simulink model "lab2"  (R2022a)
settings: Solver=VariableStepAuto  StartTime=0.0  StopTime=10.0  RelTol=1e-3
settings Model: Creator=Комп  LastModifiedBy=Комп

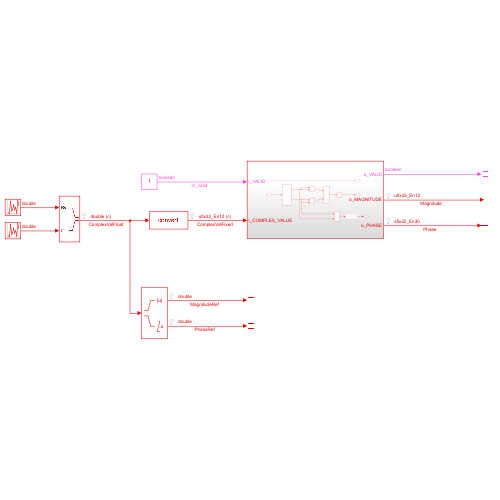
[thumbnail: Simulink's stored preview of the top-level diagram]
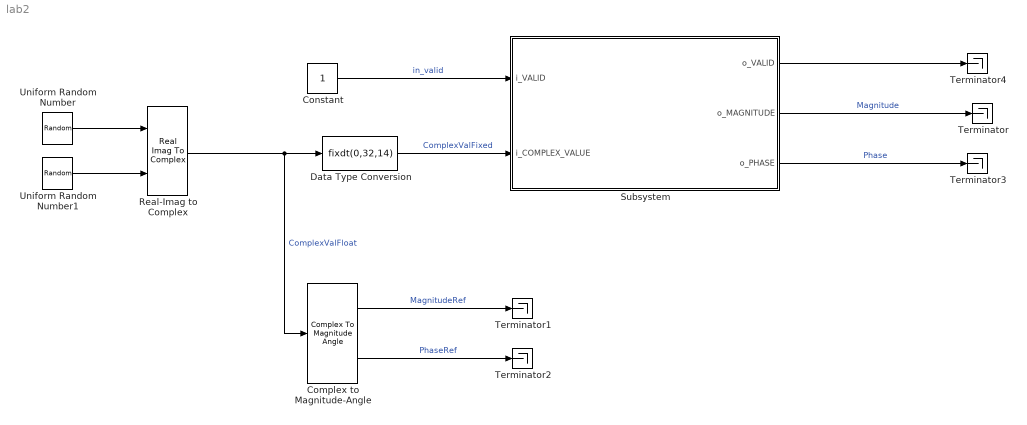
== system lab2 ==
  Complex to Magnitude-Angle : ComplexToMagnitudeAngle
  Constant : Constant  OutDataTypeStr=boolean
  Data Type Conversion : DataTypeConversion  OutDataTypeStr=fixdt(0,32,14)  RndMeth=Round  SaturateOnIntegerOverflow=off
  Real-Imag to Complex : RealImagToComplex
  Subsystem : Subsystem
  Terminator{,1..4} (5 alike) : Terminator
  Uniform Random Number : UniformRandomNumber  Minimum=0  Maximum=2^(18)-1  Seed=18  SampleTime=1
  Uniform Random Number1 : UniformRandomNumber  Minimum=0  Maximum=2^(18)-1  Seed=19  SampleTime=1
  wires:
  Uniform Random Number/1 -> Real-Imag to Complex/1
  Uniform Random Number1/1 -> Real-Imag to Complex/2
  Real-Imag to Complex/1 -> Complex to Magnitude-Angle/1, Data Type Conversion/1  "ComplexValFloat"
  Constant/1 -> Subsystem/1(i_VALID)  "in_valid"
  Data Type Conversion/1 -> Subsystem/2(i_COMPLEX_VALUE)  "ComplexValFixed"
  Subsystem/1(o_VALID) -> Terminator4/1
  Subsystem/2(o_MAGNITUDE) -> Terminator/1  "Magnitude"
  Subsystem/3(o_PHASE) -> Terminator3/1  "Phase"
  Complex to Magnitude-Angle/1 -> Terminator1/1  "MagnitudeRef"
  Complex to Magnitude-Angle/2 -> Terminator2/1  "PhaseRef"

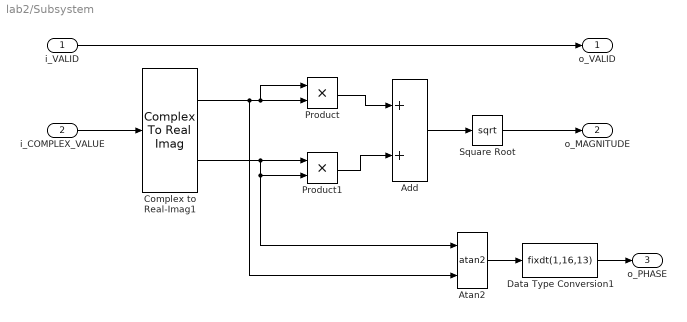
== system lab2/Subsystem ==
  i_VALID : Inport
  i_COMPLEX_VALUE : Inport  Port=2
  Add : Sum  AccumDataTypeStr=fixdt(0,65,28)  OutDataTypeStr=fixdt(0,65,28)
  Atan2 : Trigonometry  Operator=atan2  ApproximationMethod=CORDIC
  Complex to Real-Imag1 : ComplexToRealImag
  Data Type Conversion1 : DataTypeConversion  OutDataTypeStr=fixdt(1,16,13)  RndMeth=Round  SaturateOnIntegerOverflow=off
  Product : Product
  Product1 : Product
  Square Root : Sqrt  OutDataTypeStr=Inherit: Inherit via internal rule
  o_VALID : Outport
  o_MAGNITUDE : Outport  Port=2
  o_PHASE : Outport  Port=3
  wires:
  i_VALID/1 -> o_VALID/1
  Complex to Real-Imag1/2 -> Atan2/1, Product1/2, Product1/1
  Add/1 -> Square Root/1
  Complex to Real-Imag1/1 -> Atan2/2, Product/1, Product/2
  Product/1 -> Add/1
  Product1/1 -> Add/2
  i_COMPLEX_VALUE/1 -> Complex to Real-Imag1/1
  Square Root/1 -> o_MAGNITUDE/1
  Atan2/1 -> Data Type Conversion1/1
  Data Type Conversion1/1 -> o_PHASE/1
